simulink model "automata_learning"  (Simulink 10.3)
settings: Solver=VariableStepAuto  StartTime=0.0  StopTime=10.0  RelTol=1e-3
settings Model: Creator=diego  LastModifiedBy=diego
settings SolverCC: AlgebraicLoopSolver=Auto
settings DataIOCC: SaveFormat=Dataset  SignalLoggingSaveFormat=Dataset  ReturnWorkspaceOutputs=on
settings OptimizationCC: ExpressionDepthLimit=128  LifeSpan=auto
settings DebuggingCC: UnderspecifiedInitializationDetection=Simplified  MergeDetectMultiDrivingBlocksExec=error  FcnCallInpInsideContextMsg=error  StateNameClashWarn=none  SFUnexpectedBacktrackingDiag=error  SFNoUnconditionalDefaultTransitionDiag=error  SFExecutionAtInitializationDiag=warning  SFMachineParentedDataDiag=error  ArithmeticOperatorsInVariantConditions=error
settings HardwareCC: ProdBitPerPointer=64  ProdBitPerSizeT=64  ProdBitPerPtrDiffT=64  ProdLargestAtomicFloat=Float  ProdIntDivRoundTo=Zero  ProdEndianess=LittleEndian  ProdWordSize=64  ProdHWDeviceType=Intel->x86-64 (Windows64)
settings ModelReferenceCC: PropagateSignalLabelsOutOfModel=on
settings SFSimCC: SimUseLocalCustomCode=on  CustomCodeUndefinedFunction=FilterOut
settings RTWCC: RTWUseLocalCustomCode=on
settings CodeAppCC: StateflowObjectComments=off
settings GRTTargetCC: TargetLangStandard=C99 (ISO)  CombineOutputUpdateFcns=on  GRTInterface=off
settings ConfigComp: CovMetricSettings=dwe  CovSaveCumulativeToWorkspaceVar=off  CovSaveSingleToWorkspaceVar=off  CovExternalEMLEnable=on

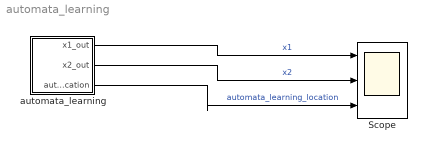
== system automata_learning ==
  Scope : Scope  NumInputPorts=3
  automata_learning : Stateflow chart  TreatAsAtomicUnit=on
  wires:
  automata_learning/1(x1_out) -> Scope/1  "x1"
  automata_learning/2(x2_out) -> Scope/2  "x2"
  automata_learning/3(automata_learning_location) -> Scope/3  "automata_learning_location"

== stateflow chart automata_learning ==
  settings: updateMethod=CONTINUOUS
  state loc1
    du:
    x1_dot = 0.4716027081012726 * (exp(0.4902026057243347 * x1 + 0.32916778326034546 * x2 + 0.12436557561159134) - 1.0) / (exp(0.4902026057243347 * x1 + 0.32916778326034546 * x2 + 0.12436557561159134) + 1.0) + 0.0772303119301796 * (exp(0.8932012319564819 * x1 + 0.4008401334285736 * x2 + 0.030844243243336678) - 1.0) / (exp(0.8932012319564819 * x1 + 0.4008401334285736 * x2 + 0.030844243243336678) + 1.0) + 0.20239026844501495 * (exp(0.031221142038702965 * x1 + 0.9505487084388733 * x2 + 0.11231078207492828) - 1.0) / (exp(0.031221142038702965 * x1 + 0.9505487084388733 * x2 + 0.11231078207492828) + 1.0) + 0.17995257675647736 * (exp(0.017666250467300415 * x2 - 0.10346487909555435 * x1 + 0.12575627863407135) - 1.0) / (exp(0.017666250467300415 * x2 - 0.10346487909555435 * x1 + 0.12575627863407135) + 1.0) - 0.14806684851646423 * (exp(0.25262296199798584 * x1 + 0.17212943732738495 * x2 - 0.09156552702188492) - 1.0) / (exp(0.25262296199798584 * x1 + 0.17212943732738495 * x2 - 0.09156552702188492) + 1.0) + 0.17653384804725647 * (exp(0.6292319893836975 * x1 - 0.7034559845924377 * x2 + 0.1486000269651413) - 1.0) / (exp(0.6292319893836975 * x1 - 0.7034559845924377 * x2 + 0.1486000269651413) + 1.0) + 0.14621903002262115 * (exp(0.35173696279525757 * x2 - 0.14781907200813293 * x1 + 0.1613396853208542) - 1.0) / (exp(0.35173696279525757 * x2 - 0.14781907200813293 * x1 + 0.1613396853208542) + 1.0) + 0.3868248462677002 * (exp(0.10623868554830551 * x1 + 0.1389903575181961 * x2 + 0.1495380848646164) - 1.0) / (exp(0.10623868554830551 * x1 + 0.1389903575181961 * x2 + 0.1495380848646164) + 1.0) + 0.026621397584676743 * (exp(0.39851248264312744 * x2 - 0.14845803380012512 * x1 + 0.1541692018508911) - 1.0) / (exp(0.39851248264312744 * x2 - 0.14845803380012512 * x1 + 0.1541692018508911) + 1.0) + 0.15215443074703217 * (exp(0.3355456292629242 * x2 - 0.17812775075435638 * x1 + 0.16218087077140808) - 1.0) / (exp(0.3355456292629242 * x2 - 0.17812775075435638 * x1 + 0.16218087077140808) + 1.0) + 0.2423621267080307 * (exp(0.31845834851264954 * x1 - 0.368916779756546 * x2 + 0.16457311809062958) - 1.0) / (exp(0.31845834851264954 * x1 - 0.368916779756546 * x2 + 0.16457311809062958) + 1.0) + 0.5095053315162659 * (exp(0.7398536205291748 * x1 + 0.5999785661697388 * x2 + 0.08746011555194855) - 1.0) / (exp(0.7398536205291748 * x1 + 0.5999785661697388 * x2 + 0.08746011555194855) + 1.0) + 0.22363349795341492 * (exp(0.4696442782878876 * x2 - 0.07120081037282944 * x1 + 0.016863320022821426) - 1.0) / (exp(0.4696442782878876 * x2 - 0.07120081037282944 * x1 + 0.016863320022821426) + 1.0) - 0.19803039729595184 * (exp(0.9458767771720886 * x2 - 0.26440635323524475 * x1 + 0.07780730724334717) - 1.0) / (exp(0.9458767771720886 * x2 - 0.26440635323524475 * x1 + 0.07780730724334717) + 1.0) + 0.10493353754281998 * (exp(0.538952648639679 * x1 - 0.04519592225551605 * x2 + 0.10528528690338135) - 1.0) / (exp(0.538952648639679 * x1 - 0.04519592225551605 * x2 + 0.10528528690338135) + 1.0) + 0.1281740963459015 * (exp(0.40728944540023804 * x2 - 0.03385405242443085 * x1 + 0.024185331538319588) - 1.0) / (exp(0.40728944540023804 * x2 - 0.03385405242443085 * x1 + 0.024185331538319588) + 1.0) + 0.1877327561378479 * (exp(0.44407951831817627 * x1 + 0.0875476822257042 * x2 + 0.13712674379348755) - 1.0) / (exp(0.44407951831817627 * x1 + 0.0875476822257042 * x2 + 0.13712674379348755) + 1.0) + 0.5150861144065857 * (exp(0.6719331741333008 * x2 - 0.22213947772979736 * x1 + 0.15428362786769867) - 1.0) / (exp(0.6719331741333008 * x2 - 0.22213947772979736 * x1 + 0.15428362786769867) + 1.0) - 0.3226105272769928 * (exp(0.29101788997650146 * x1 + 0.20947115123271942 * x2 - 0.10489220917224884) - 1.0) / (exp(0.29101788997650146 * x1 + 0.20947115123271942 * x2 - 0.10489220917224884) + 1.0) + 0.4981163442134857 * (exp(0.37576398253440857 * x1 + 0.5992299318313599 * x2 + 0.11554664373397827) - 1.0) / (exp(0.37576398253440857 * x1 + 0.5992299318313599 * x2 + 0.11554664373397827) + 1.0) + 0.0695658028125763 * (exp(0.3645703196525574 * x1 + 0.4950220584869385 * x2 + 0.07197729498147964) - 1.0) / (exp(0.3645703196525574 * x1 + 0.4950220584869385 * x2 + 0.07197729498147964) + 1.0) + 0.13338574767112732 * (exp(0.166144460439682 * x1 - 0.7433528900146484 * x2 + 0.112460657954216) - 1.0) / (exp(0.166144460439682 * x1 - 0.7433528900146484 * x2 + 0.112460657954216) + 1.0) - 0.06897702813148499 * (exp(0.41647300124168396 * x1 + 0.050582122057676315 * x2 - 0.08496729284524918) - 1.0) / (exp(0.41647300124168396 * x1 + 0.050582122057676315 * x2 - 0.08496729284524918) + 1.0) - 0.05625724419951439 * (exp(0.24224448204040527 * x1 + 0.839276909828186 * x2 - 0.06872670352458954) - 1.0) / (exp(0.24224448204040527 * x1 + 0.839276909828186 * x2 - 0.06872670352458954) + 1.0) - 0.30314353108406067 * (exp(0.3862956762313843 * x1 - 0.330698162317276 * x2 + 0.029494404792785645) - 1.0) / (exp(0.3862956762313843 * x1 - 0.330698162317276 * x2 + 0.029494404792785645) + 1.0) - 0.31301164627075195 * (exp(0.20147834718227386 * x1 + 0.7627087831497192 * x2 - 0.10361041128635406) - 1.0) / (exp(0.20147834718227386 * x1 + 0.7627087831497192 * x2 - 0.10361041128635406) + 1.0) + 0.06647036969661713 * (exp(0.09352666139602661 * x2 - 0.4191778898239136 * x1 + 0.050854817032814026) - 1.0) / (exp(0.09352666139602661 * x2 - 0.4191778898239136 * x1 + 0.050854817032814026) + 1.0) - 0.2553624212741852 * (exp(0.26251816749572754 * x1 + 0.22895655035972595 * x2 - 0.06057656556367874) - 1.0) / (exp(0.26251816749572754 * x1 + 0.22895655035972595 * x2 - 0.06057656556367874) + 1.0) - 0.2612907886505127 * (exp(0.4114644527435303 * x1 + 0.4958406686782837 * x2 - 0.07632268220186234) - 1.0) / (exp(0.4114644527435303 * x1 + 0.4958406686782837 * x2 - 0.07632268220186234) + 1.0) + 0.21924301981925964 * (exp(0.41340237855911255 * x2 - 0.6624827980995178 * x1 + 0.11923247575759888) - 1.0) / (exp(0.41340237855911255 * x2 - 0.6624827980995178 * x1 + 0.11923247575759888) + 1.0) + 0.08347097039222717;
    x2_dot = 0.29953667521476746 * (exp(0.8932012319564819 * x1 + 0.4008401334285736 * x2 + 0.030844243243336678) - 1.0) / (exp(0.8932012319564819 * x1 + 0.4008401334285736 * x2 + 0.030844243243336678) + 1.0) - 0.29886001348495483 * (exp(0.4902026057243347 * x1 + 0.32916778326034546 * x2 + 0.12436557561159134) - 1.0) / (exp(0.4902026057243347 * x1 + 0.32916778326034546 * x2 + 0.12436557561159134) + 1.0) + 0.3447601795196533 * (exp(0.031221142038702965 * x1 + 0.9505487084388733 * x2 + 0.11231078207492828) - 1.0) / (exp(0.031221142038702965 * x1 + 0.9505487084388733 * x2 + 0.11231078207492828) + 1.0) - 0.30129608511924744 * (exp(0.017666250467300415 * x2 - 0.10346487909555435 * x1 + 0.12575627863407135) - 1.0) / (exp(0.017666250467300415 * x2 - 0.10346487909555435 * x1 + 0.12575627863407135) + 1.0) + 0.3042064905166626 * (exp(0.25262296199798584 * x1 + 0.17212943732738495 * x2 - 0.09156552702188492) - 1.0) / (exp(0.25262296199798584 * x1 + 0.17212943732738495 * x2 - 0.09156552702188492) + 1.0) + 0.05604499578475952 * (exp(0.6292319893836975 * x1 - 0.7034559845924377 * x2 + 0.1486000269651413) - 1.0) / (exp(0.6292319893836975 * x1 - 0.7034559845924377 * x2 + 0.1486000269651413) + 1.0) + 0.08056741952896118 * (exp(0.35173696279525757 * x2 - 0.14781907200813293 * x1 + 0.1613396853208542) - 1.0) / (exp(0.35173696279525757 * x2 - 0.14781907200813293 * x1 + 0.1613396853208542) + 1.0) + 0.43961355090141296 * (exp(0.10623868554830551 * x1 + 0.1389903575181961 * x2 + 0.1495380848646164) - 1.0) / (exp(0.10623868554830551 * x1 + 0.1389903575181961 * x2 + 0.1495380848646164) + 1.0) + 0.21277497708797455 * (exp(0.39851248264312744 * x2 - 0.14845803380012512 * x1 + 0.1541692018508911) - 1.0) / (exp(0.39851248264312744 * x2 - 0.14845803380012512 * x1 + 0.1541692018508911) + 1.0) + 0.2397332340478897 * (exp(0.3355456292629242 * x2 - 0.17812775075435638 * x1 + 0.16218087077140808) - 1.0) / (exp(0.3355456292629242 * x2 - 0.17812775075435638 * x1 + 0.16218087077140808) + 1.0) + 0.038934774696826935 * (exp(0.31845834851264954 * x1 - 0.368916779756546 * x2 + 0.16457311809062958) - 1.0) / (exp(0.31845834851264954 * x1 - 0.368916779756546 * x2 + 0.16457311809062958) + 1.0) - 0.21872496604919434 * (exp(0.7398536205291748 * x1 + 0.5999785661697388 * x2 + 0.08746011555194855) - 1.0) / (exp(0.7398536205291748 * x1 + 0.5999785661697388 * x2 + 0.08746011555194855) + 1.0) - 0.2105134278535843 * (exp(0.4696442782878876 * x2 - 0.07120081037282944 * x1 + 0.016863320022821426) - 1.0) / (exp(0.4696442782878876 * x2 - 0.07120081037282944 * x1 + 0.016863320022821426) + 1.0) + 0.42845234274864197 * (exp(0.9458767771720886 * x2 - 0.26440635323524475 * x1 + 0.07780730724334717) - 1.0) / (exp(0.9458767771720886 * x2 - 0.26440635323524475 * x1 + 0.07780730724334717) + 1.0) - 0.07858988642692566 * (exp(0.538952648639679 * x1 - 0.04519592225551605 * x2 + 0.10528528690338135) - 1.0) / (exp(0.538952648639679 * x1 - 0.04519592225551605 * x2 + 0.10528528690338135) + 1.0) - 0.08358963578939438 * (exp(0.40728944540023804 * x2 - 0.03385405242443085 * x1 + 0.024185331538319588) - 1.0) / (exp(0.40728944540023804 * x2 - 0.03385405242443085 * x1 + 0.024185331538319588) + 1.0) + 0.22452028095722198 * (exp(0.44407951831817627 * x1 + 0.0875476822257042 * x2 + 0.13712674379348755) - 1.0) / (exp(0.44407951831817627 * x1 + 0.0875476822257042 * x2 + 0.13712674379348755) + 1.0) + 0.4255010187625885 * (exp(0.6719331741333008 * x2 - 0.22213947772979736 * x1 + 0.15428362786769867) - 1.0) / (exp(0.6719331741333008 * x2 - 0.22213947772979736 * x1 + 0.15428362786769867) + 1.0) + 0.4666166603565216 * (exp(0.29101788997650146 * x1 + 0.20947115123271942 * x2 - 0.10489220917224884) - 1.0) / (exp(0.29101788997650146 * x1 + 0.20947115123271942 * x2 - 0.10489220917224884) + 1.0) + 0.11458497494459152 * (exp(0.37576398253440857 * x1 + 0.5992299318313599 * x2 + 0.11554664373397827) - 1.0) / (exp(0.37576398253440857 * x1 + 0.5992299318313599 * x2 + 0.11554664373397827) + 1.0) + 0.4029846787452698 * (exp(0.3645703196525574 * x1 + 0.4950220584869385 * x2 + 0.07197729498147964) - 1.0) / (exp(0.3645703196525574 * x1 + 0.4950220584869385 * x2 + 0.07197729498147964) + 1.0) - 0.06546036899089813 * (exp(0.166144460439682 * x1 - 0.7433528900146484 * x2 + 0.112460657954216) - 1.0) / (exp(0.166144460439682 * x1 - 0.7433528900146484 * x2 + 0.112460657954216) + 1.0) + 0.35050633549690247 * (exp(0.41647300124168396 * x1 + 0.050582122057676315 * x2 - 0.08496729284524918) - 1.0) / (exp(0.41647300124168396 * x1 + 0.050582122057676315 * x2 - 0.08496729284524918) + 1.0) - 0.14467309415340424 * (exp(0.24224448204040527 * x1 + 0.839276909828186 * x2 - 0.06872670352458954) - 1.0) / (exp(0.24224448204040527 * x1 + 0.839276909828186 * x2 - 0.06872670352458954) + 1.0) + 0.3925016522407532 * (exp(0.3862956762313843 * x1 - 0.330698162317276 * x2 + 0.029494404792785645) - 1.0) / (exp(0.3862956762313843 * x1 - 0.330698162317276 * x2 + 0.029494404792785645) + 1.0) - 0.0077490536496043205 * (exp(0.20147834718227386 * x1 + 0.7627087831497192 * x2 - 0.10361041128635406) - 1.0) / (exp(0.20147834718227386 * x1 + 0.7627087831497192 * x2 - 0.10361041128635406) + 1.0) - 0.37136954069137573 * (exp(0.09352666139602661 * x2 - 0.4191778898239136 * x1 + 0.050854817032814026) - 1.0) / (exp(0.09352666139602661 * x2 - 0.4191778898239136 * x1 + 0.050854817032814026) + 1.0) + 0.495627224445343 * (exp(0.26251816749572754 * x1 + 0.22895655035972595 * x2 - 0.06057656556367874) - 1.0) / (exp(0.26251816749572754 * x1 + 0.22895655035972595 * x2 - 0.06057656556367874) + 1.0) + 0.30337753891944885 * (exp(0.4114644527435303 * x1 + 0.4958406686782837 * x2 - 0.07632268220186234) - 1.0) / (exp(0.4114644527435303 * x1 + 0.4958406686782837 * x2 - 0.07632268220186234) + 1.0) - 0.1606845110654831 * (exp(0.41340237855911255 * x2 - 0.6624827980995178 * x1 + 0.11923247575759888) - 1.0) / (exp(0.41340237855911255 * x2 - 0.6624827980995178 * x1 + 0.11923247575759888) + 1.0) + 0.06921185553073883;
    x1_out=x1;
    x2_out=x2;
    automata_learning_location =1;
  state loc2
    du:
    x1_dot = 0.09940944612026215 * (exp(0.5129854679107666 * x1 - 0.18030770123004913 * x2 + 0.1873820722103119) - 1.0) / (exp(0.5129854679107666 * x1 - 0.18030770123004913 * x2 + 0.1873820722103119) + 1.0) - 0.42218178510665894 * (exp(0.6277164220809937 * x1 + 0.617414116859436 * x2 + 0.004451151471585035) - 1.0) / (exp(0.6277164220809937 * x1 + 0.617414116859436 * x2 + 0.004451151471585035) + 1.0) - 0.3160305321216583 * (exp(0.08397187292575836 * x2 - 0.2538594901561737 * x1 + 0.16200947761535645) - 1.0) / (exp(0.08397187292575836 * x2 - 0.2538594901561737 * x1 + 0.16200947761535645) + 1.0) - 0.39030373096466064 * (exp(0.36400753259658813 * x1 + 0.15067961812019348 * x2 + 0.13504287600517273) - 1.0) / (exp(0.36400753259658813 * x1 + 0.15067961812019348 * x2 + 0.13504287600517273) + 1.0) - 0.27643054723739624 * (exp(0.31390586495399475 * x2 - 0.6137946844100952 * x1 + 0.1702032834291458) - 1.0) / (exp(0.31390586495399475 * x2 - 0.6137946844100952 * x1 + 0.1702032834291458) + 1.0) - 0.479932963848114 * (exp(0.8240847587585449 * x2 - 0.28391969203948975 * x1 + 0.03534712642431259) - 1.0) / (exp(0.8240847587585449 * x2 - 0.28391969203948975 * x1 + 0.03534712642431259) + 1.0) - 0.16250859200954437 * (exp(0.5600892305374146 * x1 + 0.8643016815185547 * x2 + 0.0000672234091325663) - 1.0) / (exp(0.5600892305374146 * x1 + 0.8643016815185547 * x2 + 0.0000672234091325663) + 1.0) - 0.29141247272491455 * (exp(0.9385667443275452 * x1 - 0.11919985711574554 * x2 + 0.18359696865081787) - 1.0) / (exp(0.9385667443275452 * x1 - 0.11919985711574554 * x2 + 0.18359696865081787) + 1.0) - 0.03527059406042099 * (exp(0.2679094076156616 * x1 - 0.4687827527523041 * x2 + 0.06531378626823425) - 1.0) / (exp(0.2679094076156616 * x1 - 0.4687827527523041 * x2 + 0.06531378626823425) + 1.0) + 0.09653474390506744 * (exp(0.14174817502498627 * x1 + 0.6471890807151794 * x2 - 0.0032111676409840584) - 1.0) / (exp(0.14174817502498627 * x1 + 0.6471890807151794 * x2 - 0.0032111676409840584) + 1.0) + 0.014543856494128704 * (exp(0.7148066759109497 * x1 + 0.32383447885513306 * x2 - 0.005282739643007517) - 1.0) / (exp(0.7148066759109497 * x1 + 0.32383447885513306 * x2 - 0.005282739643007517) + 1.0) - 0.31576135754585266 * (exp(0.7772475481033325 * x1 + 0.6205030679702759 * x2 + 0.0026706208009272814) - 1.0) / (exp(0.7772475481033325 * x1 + 0.6205030679702759 * x2 + 0.0026706208009272814) + 1.0) - 0.07309793680906296 * (exp(0.3710882067680359 * x1 + 0.42241641879081726 * x2 + 0.008037357591092587) - 1.0) / (exp(0.3710882067680359 * x1 + 0.42241641879081726 * x2 + 0.008037357591092587) + 1.0) - 0.11157591640949249 * (exp(0.8755472302436829 * x1 + 0.016193941235542297 * x2 + 0.045251455157995224) - 1.0) / (exp(0.8755472302436829 * x1 + 0.016193941235542297 * x2 + 0.045251455157995224) + 1.0) - 0.27048492431640625 * (exp(0.7174910306930542 * x2 - 0.020182371139526367 * x1 + 0.01213579811155796) - 1.0) / (exp(0.7174910306930542 * x2 - 0.020182371139526367 * x1 + 0.01213579811155796) + 1.0) + 0.21859526634216309 * (exp(0.3823607265949249 * x1 + 0.011211603879928589 * x2 - 0.17011186480522156) - 1.0) / (exp(0.3823607265949249 * x1 + 0.011211603879928589 * x2 - 0.17011186480522156) + 1.0) - 0.5246142148971558 * (exp(0.6425513029098511 * x1 + 0.8145269751548767 * x2 + 0.00035174659569747746) - 1.0) / (exp(0.6425513029098511 * x1 + 0.8145269751548767 * x2 + 0.00035174659569747746) + 1.0) - 0.4463590085506439 * (exp(0.8022674918174744 * x2 - 0.40092170238494873 * x1 + 0.01813332922756672) - 1.0) / (exp(0.8022674918174744 * x2 - 0.40092170238494873 * x1 + 0.01813332922756672) + 1.0) - 0.15713675320148468 * (exp(0.17945900559425354 * x1 + 0.018578974530100822 * x2 + 0.23023265600204468) - 1.0) / (exp(0.17945900559425354 * x1 + 0.018578974530100822 * x2 + 0.23023265600204468) + 1.0) - 0.30604884028434753 * (exp(0.9907521605491638 * x1 - 0.07089634984731674 * x2 + 0.17325547337532043) - 1.0) / (exp(0.9907521605491638 * x1 - 0.07089634984731674 * x2 + 0.17325547337532043) + 1.0) - 0.3188997805118561 * (exp(0.6597588062286377 * x2 - 0.30360668897628784 * x1 + 0.062151532620191574) - 1.0) / (exp(0.6597588062286377 * x2 - 0.30360668897628784 * x1 + 0.062151532620191574) + 1.0) - 0.0603540763258934 * (exp(0.015293381176888943 * x1 + 0.6490828394889832 * x2 + 0.0006276756757870317) - 1.0) / (exp(0.015293381176888943 * x1 + 0.6490828394889832 * x2 + 0.0006276756757870317) + 1.0) - 0.31608855724334717 * (exp(0.4966748356819153 * x2 - 0.35509493947029114 * x1 + 0.14687995612621307) - 1.0) / (exp(0.4966748356819153 * x2 - 0.35509493947029114 * x1 + 0.14687995612621307) + 1.0) - 0.3006037771701813 * (exp(0.822778046131134 * x1 + 0.5731481909751892 * x2 + 0.003578938776627183) - 1.0) / (exp(0.822778046131134 * x1 + 0.5731481909751892 * x2 + 0.003578938776627183) + 1.0) - 0.10746271908283234 * (exp(0.9494896531105042 * x1 - 0.31396573781967163 * x2 + 0.18377900123596191) - 1.0) / (exp(0.9494896531105042 * x1 - 0.31396573781967163 * x2 + 0.18377900123596191) + 1.0) + 0.12556539475917816 * (exp(0.8368351459503174 * x1 + 0.7917801737785339 * x2 - 0.00008519824041286483) - 1.0) / (exp(0.8368351459503174 * x1 + 0.7917801737785339 * x2 - 0.00008519824041286483) + 1.0) - 0.3539440929889679 * (exp(0.11118344217538834 * x1 + 0.40518802404403687 * x2 + 0.07945182919502258) - 1.0) / (exp(0.11118344217538834 * x1 + 0.40518802404403687 * x2 + 0.07945182919502258) + 1.0) - 0.09993302077054977 * (exp(0.48451855778694153 * x1 + 0.3026280701160431 * x2 + 0.024994682520627975) - 1.0) / (exp(0.48451855778694153 * x1 + 0.3026280701160431 * x2 + 0.024994682520627975) + 1.0) - 0.047244176268577576 * (exp(0.4798101484775543 * x1 + 0.23761166632175446 * x2 - 0.002144238678738475) - 1.0) / (exp(0.4798101484775543 * x1 + 0.23761166632175446 * x2 - 0.002144238678738475) + 1.0) - 0.5185962319374084 * (exp(0.4929291903972626 * x1 + 0.5782368779182434 * x2 + 0.014680703170597553) - 1.0) / (exp(0.4929291903972626 * x1 + 0.5782368779182434 * x2 + 0.014680703170597553) + 1.0) - 0.0967850461602211;
    x2_dot = 0.33681049942970276 * (exp(0.9385667443275452 * x1 - 0.11919985711574554 * x2 + 0.18359696865081787) - 1.0) / (exp(0.9385667443275452 * x1 - 0.11919985711574554 * x2 + 0.18359696865081787) + 1.0) + 0.14419449865818024 * (exp(0.6277164220809937 * x1 + 0.617414116859436 * x2 + 0.004451151471585035) - 1.0) / (exp(0.6277164220809937 * x1 + 0.617414116859436 * x2 + 0.004451151471585035) + 1.0) - 0.38718295097351074 * (exp(0.08397187292575836 * x2 - 0.2538594901561737 * x1 + 0.16200947761535645) - 1.0) / (exp(0.08397187292575836 * x2 - 0.2538594901561737 * x1 + 0.16200947761535645) + 1.0) - 0.09114948660135269 * (exp(0.36400753259658813 * x1 + 0.15067961812019348 * x2 + 0.13504287600517273) - 1.0) / (exp(0.36400753259658813 * x1 + 0.15067961812019348 * x2 + 0.13504287600517273) + 1.0) + 0.06673061847686768 * (exp(0.31390586495399475 * x2 - 0.6137946844100952 * x1 + 0.1702032834291458) - 1.0) / (exp(0.31390586495399475 * x2 - 0.6137946844100952 * x1 + 0.1702032834291458) + 1.0) + 0.4028923809528351 * (exp(0.8240847587585449 * x2 - 0.28391969203948975 * x1 + 0.03534712642431259) - 1.0) / (exp(0.8240847587585449 * x2 - 0.28391969203948975 * x1 + 0.03534712642431259) + 1.0) - 0.0999240130186081 * (exp(0.5600892305374146 * x1 + 0.8643016815185547 * x2 + 0.0000672234091325663) - 1.0) / (exp(0.5600892305374146 * x1 + 0.8643016815185547 * x2 + 0.0000672234091325663) + 1.0) + 0.37331923842430115 * (exp(0.5129854679107666 * x1 - 0.18030770123004913 * x2 + 0.1873820722103119) - 1.0) / (exp(0.5129854679107666 * x1 - 0.18030770123004913 * x2 + 0.1873820722103119) + 1.0) + 0.3410731852054596 * (exp(0.2679094076156616 * x1 - 0.4687827527523041 * x2 + 0.06531378626823425) - 1.0) / (exp(0.2679094076156616 * x1 - 0.4687827527523041 * x2 + 0.06531378626823425) + 1.0) - 0.25230082869529724 * (exp(0.14174817502498627 * x1 + 0.6471890807151794 * x2 - 0.0032111676409840584) - 1.0) / (exp(0.14174817502498627 * x1 + 0.6471890807151794 * x2 - 0.0032111676409840584) + 1.0) - 0.12504620850086212 * (exp(0.7148066759109497 * x1 + 0.32383447885513306 * x2 - 0.005282739643007517) - 1.0) / (exp(0.7148066759109497 * x1 + 0.32383447885513306 * x2 - 0.005282739643007517) + 1.0) - 0.14907056093215942 * (exp(0.7772475481033325 * x1 + 0.6205030679702759 * x2 + 0.0026706208009272814) - 1.0) / (exp(0.7772475481033325 * x1 + 0.6205030679702759 * x2 + 0.0026706208009272814) + 1.0) + 0.2956780791282654 * (exp(0.3710882067680359 * x1 + 0.42241641879081726 * x2 + 0.008037357591092587) - 1.0) / (exp(0.3710882067680359 * x1 + 0.42241641879081726 * x2 + 0.008037357591092587) + 1.0) + 0.3950228691101074 * (exp(0.8755472302436829 * x1 + 0.016193941235542297 * x2 + 0.045251455157995224) - 1.0) / (exp(0.8755472302436829 * x1 + 0.016193941235542297 * x2 + 0.045251455157995224) + 1.0) + 0.49911952018737793 * (exp(0.7174910306930542 * x2 - 0.020182371139526367 * x1 + 0.01213579811155796) - 1.0) / (exp(0.7174910306930542 * x2 - 0.020182371139526367 * x1 + 0.01213579811155796) + 1.0) - 0.1835329383611679 * (exp(0.3823607265949249 * x1 + 0.011211603879928589 * x2 - 0.17011186480522156) - 1.0) / (exp(0.3823607265949249 * x1 + 0.011211603879928589 * x2 - 0.17011186480522156) + 1.0) + 0.42436978220939636 * (exp(0.6425513029098511 * x1 + 0.8145269751548767 * x2 + 0.00035174659569747746) - 1.0) / (exp(0.6425513029098511 * x1 + 0.8145269751548767 * x2 + 0.00035174659569747746) + 1.0) - 0.3059418499469757 * (exp(0.8022674918174744 * x2 - 0.40092170238494873 * x1 + 0.01813332922756672) - 1.0) / (exp(0.8022674918174744 * x2 - 0.40092170238494873 * x1 + 0.01813332922756672) + 1.0) + 0.2961410880088806 * (exp(0.17945900559425354 * x1 + 0.018578974530100822 * x2 + 0.23023265600204468) - 1.0) / (exp(0.17945900559425354 * x1 + 0.018578974530100822 * x2 + 0.23023265600204468) + 1.0) + 0.24017132818698883 * (exp(0.9907521605491638 * x1 - 0.07089634984731674 * x2 + 0.17325547337532043) - 1.0) / (exp(0.9907521605491638 * x1 - 0.07089634984731674 * x2 + 0.17325547337532043) + 1.0) - 0.1033150926232338 * (exp(0.6597588062286377 * x2 - 0.30360668897628784 * x1 + 0.062151532620191574) - 1.0) / (exp(0.6597588062286377 * x2 - 0.30360668897628784 * x1 + 0.062151532620191574) + 1.0) + 0.0581403486430645 * (exp(0.015293381176888943 * x1 + 0.6490828394889832 * x2 + 0.0006276756757870317) - 1.0) / (exp(0.015293381176888943 * x1 + 0.6490828394889832 * x2 + 0.0006276756757870317) + 1.0) + 0.22430425882339478 * (exp(0.4966748356819153 * x2 - 0.35509493947029114 * x1 + 0.14687995612621307) - 1.0) / (exp(0.4966748356819153 * x2 - 0.35509493947029114 * x1 + 0.14687995612621307) + 1.0) + 0.04207557439804077 * (exp(0.822778046131134 * x1 + 0.5731481909751892 * x2 + 0.003578938776627183) - 1.0) / (exp(0.822778046131134 * x1 + 0.5731481909751892 * x2 + 0.003578938776627183) + 1.0) + 0.28885316848754883 * (exp(0.9494896531105042 * x1 - 0.31396573781967163 * x2 + 0.18377900123596191) - 1.0) / (exp(0.9494896531105042 * x1 - 0.31396573781967163 * x2 + 0.18377900123596191) + 1.0) - 0.16381853818893433 * (exp(0.8368351459503174 * x1 + 0.7917801737785339 * x2 - 0.00008519824041286483) - 1.0) / (exp(0.8368351459503174 * x1 + 0.7917801737785339 * x2 - 0.00008519824041286483) + 1.0) - 0.19841310381889343 * (exp(0.11118344217538834 * x1 + 0.40518802404403687 * x2 + 0.07945182919502258) - 1.0) / (exp(0.11118344217538834 * x1 + 0.40518802404403687 * x2 + 0.07945182919502258) + 1.0) - 0.1740700751543045 * (exp(0.48451855778694153 * x1 + 0.3026280701160431 * x2 + 0.024994682520627975) - 1.0) / (exp(0.48451855778694153 * x1 + 0.3026280701160431 * x2 + 0.024994682520627975) + 1.0) + 0.18555928766727448 * (exp(0.4798101484775543 * x1 + 0.23761166632175446 * x2 - 0.002144238678738475) - 1.0) / (exp(0.4798101484775543 * x1 + 0.23761166632175446 * x2 - 0.002144238678738475) + 1.0) - 0.13522174954414368 * (exp(0.4929291903972626 * x1 + 0.5782368779182434 * x2 + 0.014680703170597553) - 1.0) / (exp(0.4929291903972626 * x1 + 0.5782368779182434 * x2 + 0.014680703170597553) + 1.0) + 0.08975403755903244;
    x1_out=x1;
    x2_out=x2;
    automata_learning_location =2;
  state loc3
    du:
    x1_dot = 0.13391880691051483 * (exp(0.06181495264172554 * x1 + 0.830928385257721 * x2 - 0.00042180376476608217) - 1.0) / (exp(0.06181495264172554 * x1 + 0.830928385257721 * x2 - 0.00042180376476608217) + 1.0) - 0.11919530481100082 * (exp(0.522223949432373 * x1 - 0.6981194615364075 * x2 + 0.002108635613694787) - 1.0) / (exp(0.522223949432373 * x1 - 0.6981194615364075 * x2 + 0.002108635613694787) + 1.0) + 0.19859743118286133 * (exp(0.5409014225006104 * x1 - 0.18676605820655823 * x2 + 0.1448603719472885) - 1.0) / (exp(0.5409014225006104 * x1 - 0.18676605820655823 * x2 + 0.1448603719472885) + 1.0) + 0.015296559780836105 * (exp(0.5186636447906494 * x1 - 0.7686441540718079 * x2 + 0.0011455173371359706) - 1.0) / (exp(0.5186636447906494 * x1 - 0.7686441540718079 * x2 + 0.0011455173371359706) + 1.0) - 0.4283091127872467 * (exp(0.5837187170982361 * x1 + 0.4516241252422333 * x2 - 0.03196272999048233) - 1.0) / (exp(0.5837187170982361 * x1 + 0.4516241252422333 * x2 - 0.03196272999048233) + 1.0) + 0.3406931161880493 * (exp(0.676913857460022 * x1 + 0.5504132509231567 * x2 - 0.006321039516478777) - 1.0) / (exp(0.676913857460022 * x1 + 0.5504132509231567 * x2 - 0.006321039516478777) + 1.0) + 0.3375319838523865 * (exp(0.7741734385490417 * x2 - 0.15453040599822998 * x1 + 0.000163470976985991) - 1.0) / (exp(0.7741734385490417 * x2 - 0.15453040599822998 * x1 + 0.000163470976985991) + 1.0) + 0.09929674118757248 * (exp(0.38023465871810913 * x1 - 0.726379930973053 * x2 + 0.00029279489535838366) - 1.0) / (exp(0.38023465871810913 * x1 - 0.726379930973053 * x2 + 0.00029279489535838366) + 1.0) - 0.09152176231145859 * (exp(0.7769408226013184 * x2 - 0.16671495139598846 * x1 + 0.0012986381771042943) - 1.0) / (exp(0.7769408226013184 * x2 - 0.16671495139598846 * x1 + 0.0012986381771042943) + 1.0) + 0.057577308267354965 * (exp(0.6970188021659851 * x2 - 0.2001141607761383 * x1 + 0.004786035045981407) - 1.0) / (exp(0.6970188021659851 * x2 - 0.2001141607761383 * x1 + 0.004786035045981407) + 1.0) - 0.12983807921409607 * (exp(0.8190765976905823 * x1 + 0.19012735784053802 * x2 + 0.13562315702438354) - 1.0) / (exp(0.8190765976905823 * x1 + 0.19012735784053802 * x2 + 0.13562315702438354) + 1.0) + 0.31065547466278076 * (exp(0.7990989089012146 * x1 + 0.09012157469987869 * x2 - 0.15513083338737488) - 1.0) / (exp(0.7990989089012146 * x1 + 0.09012157469987869 * x2 - 0.15513083338737488) + 1.0) + 0.3659955859184265 * (exp(0.23125216364860535 * x1 + 0.6959024667739868 * x2 + 0.00012704286200460047) - 1.0) / (exp(0.23125216364860535 * x1 + 0.6959024667739868 * x2 + 0.00012704286200460047) + 1.0) - 0.20614756643772125 * (exp(0.18442755937576294 * x1 + 0.2617461681365967 * x2 + 0.11357703059911728) - 1.0) / (exp(0.18442755937576294 * x1 + 0.2617461681365967 * x2 + 0.11357703059911728) + 1.0) - 0.423560231924057 * (exp(0.735741138458252 * x1 + 0.45589232444763184 * x2 - 0.016892028972506523) - 1.0) / (exp(0.735741138458252 * x1 + 0.45589232444763184 * x2 - 0.016892028972506523) + 1.0) - 0.00873386487364769 * (exp(0.4189932346343994 * x1 + 0.08070419728755951 * x2 + 0.18171867728233337) - 1.0) / (exp(0.4189932346343994 * x1 + 0.08070419728755951 * x2 + 0.18171867728233337) + 1.0) + 0.2383020669221878 * (exp(0.6878048181533813 * x2 - 0.7323256731033325 * x1 + 0.00617991155013442) - 1.0) / (exp(0.6878048181533813 * x2 - 0.7323256731033325 * x1 + 0.00617991155013442) + 1.0) - 0.42847388982772827 * (exp(0.2325640171766281 * x2 - 0.6580464243888855 * x1 + 0.07914160192012787) - 1.0) / (exp(0.2325640171766281 * x2 - 0.6580464243888855 * x1 + 0.07914160192012787) + 1.0) - 0.08512790501117706 * (exp(0.6077308654785156 * x1 + 0.7174503803253174 * x2 + 0.0036251882556825876) - 1.0) / (exp(0.6077308654785156 * x1 + 0.7174503803253174 * x2 + 0.0036251882556825876) + 1.0) - 0.11688737571239471 * (exp(0.8507214188575745 * x2 - 0.4046079218387604 * x1 + 0.0005854947958141565) - 1.0) / (exp(0.8507214188575745 * x2 - 0.4046079218387604 * x1 + 0.0005854947958141565) + 1.0) + 0.3675585389137268 * (exp(0.6745675206184387 * x1 + 0.11397437751293182 * x2 - 0.0964978039264679) - 1.0) / (exp(0.6745675206184387 * x1 + 0.11397437751293182 * x2 - 0.0964978039264679) + 1.0) + 0.21359951794147491 * (exp(0.44495517015457153 * x2 - 0.5907729864120483 * x1 + 0.05593755096197128) - 1.0) / (exp(0.44495517015457153 * x2 - 0.5907729864120483 * x1 + 0.05593755096197128) + 1.0) + 0.35291817784309387 * (exp(0.6072133183479309 * x2 - 0.8590480089187622 * x1 + 0.014273274689912796) - 1.0) / (exp(0.6072133183479309 * x2 - 0.8590480089187622 * x1 + 0.014273274689912796) + 1.0) + 0.38521742820739746 * (exp(0.8470609784126282 * x2 - 0.20842193067073822 * x1 + 0.0006987780798226595) - 1.0) / (exp(0.8470609784126282 * x2 - 0.20842193067073822 * x1 + 0.0006987780798226595) + 1.0) - 0.11519917845726013 * (exp(0.626823902130127 * x2 - 0.8023239970207214 * x1 + 0.01543375477194786) - 1.0) / (exp(0.626823902130127 * x2 - 0.8023239970207214 * x1 + 0.01543375477194786) + 1.0) - 0.2617543637752533 * (exp(0.027313269674777985 * x1 + 0.23437267541885376 * x2 - 0.07693794369697571) - 1.0) / (exp(0.027313269674777985 * x1 + 0.23437267541885376 * x2 - 0.07693794369697571) + 1.0) - 0.14551043510437012 * (exp(0.09938313066959381 * x2 - 0.7570124864578247 * x1 + 0.11116168648004532) - 1.0) / (exp(0.09938313066959381 * x2 - 0.7570124864578247 * x1 + 0.11116168648004532) + 1.0) - 0.012510816566646099 * (exp(0.7602941989898682 * x1 + 0.8424192667007446 * x2 - 0.0004436737799551338) - 1.0) / (exp(0.7602941989898682 * x1 + 0.8424192667007446 * x2 - 0.0004436737799551338) + 1.0) - 0.2714858949184418 * (exp(0.46065810322761536 * x1 + 0.806241512298584 * x2 - 0.0008009360171854496) - 1.0) / (exp(0.46065810322761536 * x1 + 0.806241512298584 * x2 - 0.0008009360171854496) + 1.0) - 0.21159721910953522 * (exp(0.24011659622192383 * x2 - 0.3292262852191925 * x1 + 0.12026399374008179) - 1.0) / (exp(0.24011659622192383 * x2 - 0.3292262852191925 * x1 + 0.12026399374008179) + 1.0) - 0.00020466868591029197;
    x2_dot = 0.24798732995986938 * (exp(0.06181495264172554 * x1 + 0.830928385257721 * x2 - 0.00042180376476608217) - 1.0) / (exp(0.06181495264172554 * x1 + 0.830928385257721 * x2 - 0.00042180376476608217) + 1.0) - 0.25351449847221375 * (exp(0.522223949432373 * x1 - 0.6981194615364075 * x2 + 0.002108635613694787) - 1.0) / (exp(0.522223949432373 * x1 - 0.6981194615364075 * x2 + 0.002108635613694787) + 1.0) - 0.2634170949459076 * (exp(0.5409014225006104 * x1 - 0.18676605820655823 * x2 + 0.1448603719472885) - 1.0) / (exp(0.5409014225006104 * x1 - 0.18676605820655823 * x2 + 0.1448603719472885) + 1.0) - 0.3005005121231079 * (exp(0.5186636447906494 * x1 - 0.7686441540718079 * x2 + 0.0011455173371359706) - 1.0) / (exp(0.5186636447906494 * x1 - 0.7686441540718079 * x2 + 0.0011455173371359706) + 1.0) + 0.32044389843940735 * (exp(0.5837187170982361 * x1 + 0.4516241252422333 * x2 - 0.03196272999048233) - 1.0) / (exp(0.5837187170982361 * x1 + 0.4516241252422333 * x2 - 0.03196272999048233) + 1.0) + 0.17418645322322845 * (exp(0.676913857460022 * x1 + 0.5504132509231567 * x2 - 0.006321039516478777) - 1.0) / (exp(0.676913857460022 * x1 + 0.5504132509231567 * x2 - 0.006321039516478777) + 1.0) - 0.03148535639047623 * (exp(0.7741734385490417 * x2 - 0.15453040599822998 * x1 + 0.000163470976985991) - 1.0) / (exp(0.7741734385490417 * x2 - 0.15453040599822998 * x1 + 0.000163470976985991) + 1.0) + 0.013643022626638412 * (exp(0.38023465871810913 * x1 - 0.726379930973053 * x2 + 0.00029279489535838366) - 1.0) / (exp(0.38023465871810913 * x1 - 0.726379930973053 * x2 + 0.00029279489535838366) + 1.0) - 0.416521817445755 * (exp(0.7769408226013184 * x2 - 0.16671495139598846 * x1 + 0.0012986381771042943) - 1.0) / (exp(0.7769408226013184 * x2 - 0.16671495139598846 * x1 + 0.0012986381771042943) + 1.0) - 0.42894044518470764 * (exp(0.6970188021659851 * x2 - 0.2001141607761383 * x1 + 0.004786035045981407) - 1.0) / (exp(0.6970188021659851 * x2 - 0.2001141607761383 * x1 + 0.004786035045981407) + 1.0) - 0.5313743352890015 * (exp(0.8190765976905823 * x1 + 0.19012735784053802 * x2 + 0.13562315702438354) - 1.0) / (exp(0.8190765976905823 * x1 + 0.19012735784053802 * x2 + 0.13562315702438354) + 1.0) + 0.2343064695596695 * (exp(0.7990989089012146 * x1 + 0.09012157469987869 * x2 - 0.15513083338737488) - 1.0) / (exp(0.7990989089012146 * x1 + 0.09012157469987869 * x2 - 0.15513083338737488) + 1.0) + 0.009861676022410393 * (exp(0.23125216364860535 * x1 + 0.6959024667739868 * x2 + 0.00012704286200460047) - 1.0) / (exp(0.23125216364860535 * x1 + 0.6959024667739868 * x2 + 0.00012704286200460047) + 1.0) - 0.36287400126457214 * (exp(0.18442755937576294 * x1 + 0.2617461681365967 * x2 + 0.11357703059911728) - 1.0) / (exp(0.18442755937576294 * x1 + 0.2617461681365967 * x2 + 0.11357703059911728) + 1.0) + 0.042243316769599915 * (exp(0.735741138458252 * x1 + 0.45589232444763184 * x2 - 0.016892028972506523) - 1.0) / (exp(0.735741138458252 * x1 + 0.45589232444763184 * x2 - 0.016892028972506523) + 1.0) - 0.3669668138027191 * (exp(0.4189932346343994 * x1 + 0.08070419728755951 * x2 + 0.18171867728233337) - 1.0) / (exp(0.4189932346343994 * x1 + 0.08070419728755951 * x2 + 0.18171867728233337) + 1.0) - 0.4460239112377167 * (exp(0.6878048181533813 * x2 - 0.7323256731033325 * x1 + 0.00617991155013442) - 1.0) / (exp(0.6878048181533813 * x2 - 0.7323256731033325 * x1 + 0.00617991155013442) + 1.0) - 0.22172729671001434 * (exp(0.2325640171766281 * x2 - 0.6580464243888855 * x1 + 0.07914160192012787) - 1.0) / (exp(0.2325640171766281 * x2 - 0.6580464243888855 * x1 + 0.07914160192012787) + 1.0) - 0.4694260060787201 * (exp(0.6077308654785156 * x1 + 0.7174503803253174 * x2 + 0.0036251882556825876) - 1.0) / (exp(0.6077308654785156 * x1 + 0.7174503803253174 * x2 + 0.0036251882556825876) + 1.0) - 0.5004711747169495 * (exp(0.8507214188575745 * x2 - 0.4046079218387604 * x1 + 0.0005854947958141565) - 1.0) / (exp(0.8507214188575745 * x2 - 0.4046079218387604 * x1 + 0.0005854947958141565) + 1.0) + 0.11379243433475494 * (exp(0.6745675206184387 * x1 + 0.11397437751293182 * x2 - 0.0964978039264679) - 1.0) / (exp(0.6745675206184387 * x1 + 0.11397437751293182 * x2 - 0.0964978039264679) + 1.0) - 0.23656167089939117 * (exp(0.44495517015457153 * x2 - 0.5907729864120483 * x1 + 0.05593755096197128) - 1.0) / (exp(0.44495517015457153 * x2 - 0.5907729864120483 * x1 + 0.05593755096197128) + 1.0) - 0.3321789801120758 * (exp(0.6072133183479309 * x2 - 0.8590480089187622 * x1 + 0.014273274689912796) - 1.0) / (exp(0.6072133183479309 * x2 - 0.8590480089187622 * x1 + 0.014273274689912796) + 1.0) - 0.4643550217151642 * (exp(0.8470609784126282 * x2 - 0.20842193067073822 * x1 + 0.0006987780798226595) - 1.0) / (exp(0.8470609784126282 * x2 - 0.20842193067073822 * x1 + 0.0006987780798226595) + 1.0) - 0.510519802570343 * (exp(0.626823902130127 * x2 - 0.8023239970207214 * x1 + 0.01543375477194786) - 1.0) / (exp(0.626823902130127 * x2 - 0.8023239970207214 * x1 + 0.01543375477194786) + 1.0) + 0.05251113697886467 * (exp(0.027313269674777985 * x1 + 0.23437267541885376 * x2 - 0.07693794369697571) - 1.0) / (exp(0.027313269674777985 * x1 + 0.23437267541885376 * x2 - 0.07693794369697571) + 1.0) - 0.13555075228214264 * (exp(0.09938313066959381 * x2 - 0.7570124864578247 * x1 + 0.11116168648004532) - 1.0) / (exp(0.09938313066959381 * x2 - 0.7570124864578247 * x1 + 0.11116168648004532) + 1.0) + 0.2771265208721161 * (exp(0.7602941989898682 * x1 + 0.8424192667007446 * x2 - 0.0004436737799551338) - 1.0) / (exp(0.7602941989898682 * x1 + 0.8424192667007446 * x2 - 0.0004436737799551338) + 1.0) + 0.2789631485939026 * (exp(0.46065810322761536 * x1 + 0.806241512298584 * x2 - 0.0008009360171854496) - 1.0) / (exp(0.46065810322761536 * x1 + 0.806241512298584 * x2 - 0.0008009360171854496) + 1.0) - 0.42788058519363403 * (exp(0.24011659622192383 * x2 - 0.3292262852191925 * x1 + 0.12026399374008179) - 1.0) / (exp(0.24011659622192383 * x2 - 0.3292262852191925 * x1 + 0.12026399374008179) + 1.0) - 0.08952217549085617;
    x1_out=x1;
    x2_out=x2;
    automata_learning_location =3;
  loc3 -> loc1 : [-0.03057 * x1 - 0.08402 * x2 + 1.0 > 0.0]
  loc1 -> loc2 : [-0.0006553 * x1 - 0.08273 * x2 + 1.0 < 0.0]
  (default) -> loc1 : {x1 = 0.0;
      | x2 = 0.0;}
  loc2 -> loc3 : [2.337 * x1 - 0.1122 * x2 + 1.0 < 0.0]
  data: x1_out output double; x1 local double; x2_out output double; x2 local double; automata_learning_location output double
  data x1 settings: updateMethod=SF_CONTINUOUS_TIME_DATA
  data x2 settings: updateMethod=SF_CONTINUOUS_TIME_DATA
